simulink model "HubSimGenerator"  (R2020b)
settings: Solver=FixedStepAuto  StartTime=0.0  StopTime=2  FixedStep=1e-4  RelTol=1e-4
libraries: simulink x1
settings Model: Creator=Utente  LastModifiedBy=Utente
settings DataIOCC: ReturnWorkspaceOutputs=off

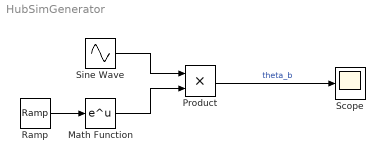
== system HubSimGenerator ==
  Math Function : Math  SaturateOnIntegerOverflow=on
  Product : Product
  Ramp : simulink/Sources/Ramp  slope=-1.22  start=0  InitialOutput=0
  Scope : Scope
  Sine Wave : Sin  Amplitude=30  Frequency=24.36948091  Phase=90  SampleTime=0
  wires:
  Math Function/1 -> Product/2
  Product/1 -> Scope/1  "theta_b"
  Sine Wave/1 -> Product/1
  Ramp/1 -> Math Function/1
